simulink model "lab2_sim"  (R2019b)
settings: Solver=ode45  StartTime=0.0  StopTime=Tfin  MaxStep=Tstep  RelTol=1e-3
values from neighbouring files (symbols this model uses):
  C = [1, 0, 0]    [lab2_prac.m]
  ref = 1    [lab2_prac.m]
  x0 = [0, 0, 0]    [lab2_prac.m]
libraries: cstblocks x1
settings Model: Creator=user  LastModifiedBy=user

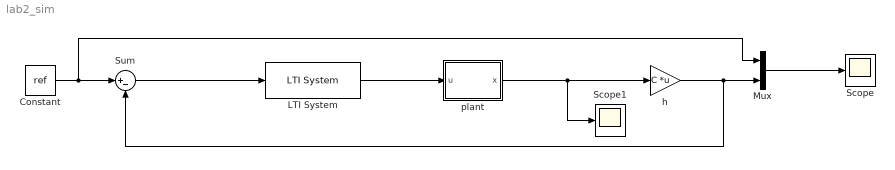
== system lab2_sim ==
  Constant : Constant  Value=ref
  LTI System : cstblocks/LTI System  sys=K  IC=[]
  Mux : Mux  Inputs=2
  Scope : Scope
  Scope1 : Scope
  Sum : Sum  Inputs=|+-
  h : Gain  Gain=C  Multiplication=Matrix(K*u)
  "plant " : Subsystem
  wires:
  "plant "/1(x) -> Scope1/1, h/1
  h/1 -> Sum/2, Mux/2
  Mux/1 -> Scope/1
  LTI System/1 -> "plant "/1(u)
  Constant/1 -> Mux/1, Sum/1
  Sum/1 -> LTI System/1

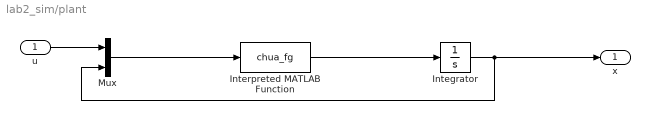
== system lab2_sim/plant  ==
  u : Inport
  Integrator : Integrator  InitialCondition=x0
  Interpreted MATLAB Function : MATLABFcn  MATLABFcn=chua_fg
  Mux : Mux  Inputs=2
  x : Outport
  wires:
  Mux/1 -> Interpreted MATLAB Function/1
  Integrator/1 -> x/1, Mux/2
  Interpreted MATLAB Function/1 -> Integrator/1
  u/1 -> Mux/1
